simulink model "forces_aero"  (R2024b)
settings: Solver=VariableStepAuto  StartTime=0.0  StopTime=10.0  RelTol=1e-3
values from neighbouring files (symbols this model uses):
  A = 1    [main_data_vehicle.m]
  CD = 0.63    [main_data_vehicle.m]
  CL = 0.29    [main_data_vehicle.m]
  rho = 1.225    [main_data_vehicle.m]
settings Model: Creator=marti  LastModifiedBy=marti

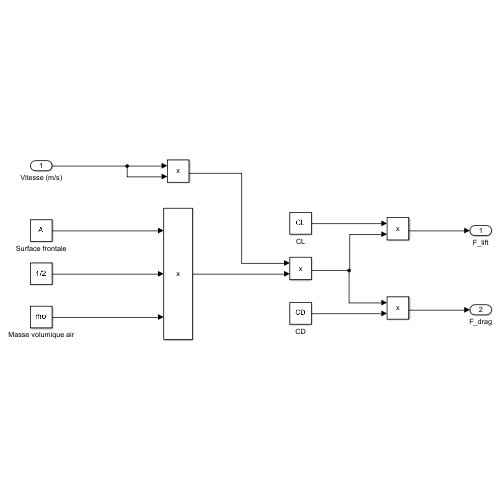
[thumbnail: Simulink's stored preview of the top-level diagram]
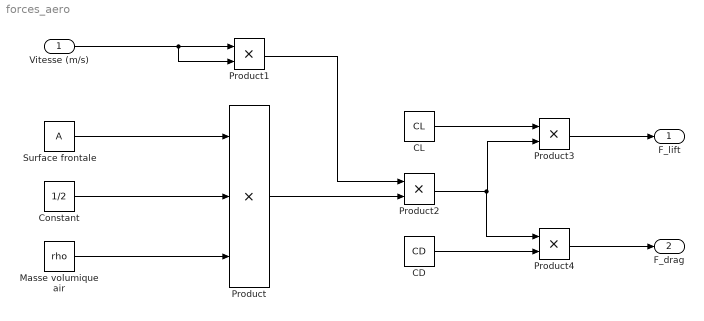
== system forces_aero ==
  Vitesse (m/s) : Inport
  CD : Constant  Value=CD
  CL : Constant  Value=CL
  Constant : Constant  Value=1/2
  Masse volumique air : Constant  Value=rho
  Product : Product  Inputs=3
  Product{1..4} (4 alike) : Product
  Surface frontale : Constant  Value=A
  F_lift : Outport
  F_drag : Outport  Port=2
  wires:
  Surface frontale/1 -> Product/1
  Masse volumique air/1 -> Product/3
  Vitesse (m/s)/1 -> Product1/2, Product1/1
  Product/1 -> Product2/2
  Constant/1 -> Product/2
  Product1/1 -> Product2/1
  CL/1 -> Product3/1
  CD/1 -> Product4/2
  Product2/1 -> Product4/1, Product3/2
  Product3/1 -> F_lift/1
  Product4/1 -> F_drag/1
